simulink model "ex_2f"  (R2016a)
settings: Solver=VariableStepAuto  StartTime=0.0  StopTime=1e6  RelTol=1e-3
libraries: simCryogenics_lib x13, nesl_utility x8
settings Model: Creator=FB229602  LastModifiedBy=FB229602
settings SimscapeCC: SimscapeLogType=all

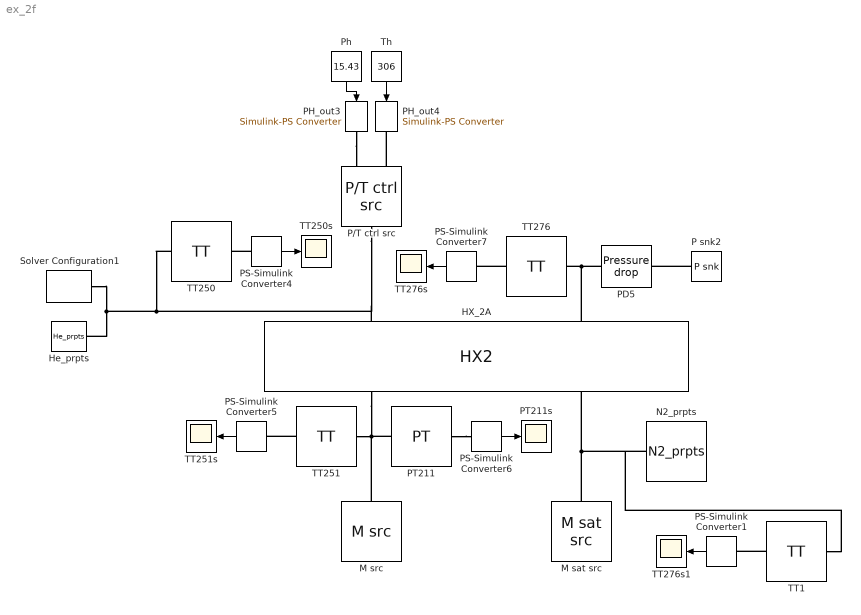
== system ex_2f ==
  HX_2A : simCryogenics_lib/Elements/HX2  N=9  Vh=1 m^3  Vc=1 m^3  M=1000 kg  Kh=0.05/0.04498 s*bar/kg  Kc=0 s*bar/kg  h=16470 J/s/K  Th0=300 K  Ph0=15 bar  Mh0=0.047 kg/s  Tc0=78 K  Pc0=1.1 bar  Mc0=0.047 kg/s
  He_prpts : simCryogenics_lib/Utilities/He_prpts  P_min=0.25 bar  T_min=3 K  T_max=320 K  P_max=20 bar  Mol=4.0026 * 10 ^ (- 3) kg/mol
  M sat src : simCryogenics_lib/Sources_Sinks/M sat src  M=0.216 kg/s  Xmix=1
  M src : simCryogenics_lib/Sources_Sinks/M src  M=0.047 kg/s
  N2_prpts : simCryogenics_lib/Utilities/N2_prpts  P_min=0.5 bar  T_min=70 K  T_max=320 K  P_max=20 bar  Mol=4.0026 * (10 ^ (- 3)) kg/mol
  P snk2 : simCryogenics_lib/Sources_Sinks/P snk  P=1.15 bar
  P/T ctrl src : simCryogenics_lib/Sources_Sinks/P//T ctrl src
  PD5 : simCryogenics_lib/Utilities/Pressure drop  K=0.05/0.216 s*bar/kg
  PH_out3 : nesl_utility/Simulink-PS Converter  PhysicalDomain=network_engine_domain  SubClassName=ps_input  LeftPortType=input  RightPortType=output  PseudoPeriodic=off  Frequencies=[]  NoiseDistribution=none  NoiseParameters=[]  Unit=bar  AffineConversion=off  InputFiltering=off  SimscapeFilterOrder=1  InputFilterTimeConstant=0.001  UdotUserProvided=1
  PH_out4 : nesl_utility/Simulink-PS Converter  PhysicalDomain=network_engine_domain  SubClassName=ps_input  LeftPortType=input  RightPortType=output  PseudoPeriodic=off  Frequencies=[]  NoiseDistribution=none  NoiseParameters=[]  Unit=K  AffineConversion=off  InputFiltering=off  SimscapeFilterOrder=1  InputFilterTimeConstant=0.001  UdotUserProvided=1
  PS-Simulink Converter{1,4..7} (5 alike) : nesl_utility/PS-Simulink Converter  PhysicalDomain=network_engine_domain  SubClassName=ps_output  LeftPortType=input  RightPortType=output  PseudoPeriodic=off  Frequencies=[]  Unit=1  AffineConversion=off
  PT211 : simCryogenics_lib/Sensors/PT
  PT211s : Scope
  Ph : Constant  Value=15.43
  Solver Configuration1 : nesl_utility/Solver Configuration  PhysicalDomain=network_engine_domain  SubClassName=solver  LeftPortType=input  RightPortType=generic  Accelerate=off  Tones=[]  Harmonics=[]  SimulateNoise=off  Profile=off  UseLocalSampling=off  EnableSwitchedLinearOptims=on  FrequencyDomain=off  UseCCode=off  RelTol=0.001  AbsTol=1e-06  MinStep=1e-09  ToWorkspace=off  RevertToSquareIcSolve=off  NumHomotopyIterations=100  PhasorMode=off  PhasorModeNumHarmonics=1  OverrideAbsTol=off  DoDC=off  ResidualTolerance=1e-09  UseLocalSolver=off  LocalSolverChoice=NE_BACKWARD_EULER_ADVANCER  LocalSolverSampleTime=20  DoFixedCost=off  MaxNonlinIter=10  MaxModeIter=2  LinearAlgebra=Sparse  DelaysMemoryBudget=1024  AutomaticFiltering=on  FilteringTimeConstant=0.001
  TT{1,250..251,276} (4 alike) : simCryogenics_lib/Sensors/TT
  TT250s : Scope
  TT251s : Scope
  TT276s : Scope
  TT276s1 : Scope
  Th : Constant  Value=306
  wires:
  PS-Simulink Converter4/1 -> TT250s/1
  PS-Simulink Converter5/1 -> TT251s/1
  PS-Simulink Converter6/1 -> PT211s/1
  PS-Simulink Converter7/1 -> TT276s/1
  Th/1 -> PH_out4/1
  Ph/1 -> PH_out3/1
  PS-Simulink Converter1/1 -> TT276s1/1
  connections:
  HX_2A/RConn2 -- M src/RConn1 -- TT251/LConn1 -- PT211/LConn1
  HX_2A/LConn1 -- PD5/LConn1 -- TT276/LConn1
  Solver Configuration1/RConn1 -- P/T ctrl src/RConn1 -- HX_2A/LConn2 -- TT250/LConn1 -- He_prpts/RConn1
  PT211/RConn1 -- PS-Simulink Converter6/LConn1
  PS-Simulink Converter4/LConn1 -- TT250/RConn1
  TT276/RConn1 -- PS-Simulink Converter7/LConn1
  P snk2/RConn1 -- PD5/RConn1
  TT251/RConn1 -- PS-Simulink Converter5/LConn1
  PH_out3/RConn1 -- P/T ctrl src/LConn1
  P/T ctrl src/LConn2 -- PH_out4/RConn1
  M sat src/RConn1 -- TT1/LConn1 -- N2_prpts/RConn1 -- HX_2A/RConn1
  TT1/RConn1 -- PS-Simulink Converter1/LConn1
